simulink model "asbQuadcopter"  (R2021b)
settings: Solver=ode3  StartTime=0  StopTime=200  FixedStep=Ts  RelTol=1e-3  EnableMultiTasking=on
undefined symbols (not defined in the file or in its folder): Command, ft, init, m, s, takeOffDuration, Ts, Vehicle
libraries: simulink x6, aerolibconvert2 x5, aerolibanimutils x3, environmentLibrary x2, SignalEditorBlockLib x2, sensorsLibrary x2, aerolibfltsims x2, aerolibutil x2, vrlib x1
settings Model: Creator=The MathWorks, Inc.  LastModifiedBy=LENOVO
settings SolverCC: AlgebraicLoopSolver=TrustRegion
settings DataIOCC: LimitDataPoints=on  SaveFormat=Array  SaveOutput=off  SignalLogging=off  DSMLogging=off  SaveTime=off  ReturnWorkspaceOutputs=off
settings OptimizationCC: BlockReduction=off  BufferReuse=off  LifeSpan=inf
settings DebuggingCC: AlgebraicLoopMsg=none  ParameterPrecisionLossMsg=none  UnconnectedInputMsg=none  UnconnectedOutputMsg=none  UnconnectedLineMsg=none  AllowSymbolicDim=off  PregeneratedLibrarySubsystemCodeDiagnostic=none  SFUnexpectedBacktrackingDiag=warning  SFNoUnconditionalDefaultTransitionDiag=warning  SFExecutionAtInitializationDiag=none  SFMachineParentedDataDiag=warning  ArithmeticOperatorsInVariantConditions=warning
settings HardwareCC: ProdBitPerPointer=32  ProdBitPerSizeT=32  ProdBitPerPtrDiffT=32  ProdLargestAtomicFloat=None  ProdIntDivRoundTo=Undefined  ProdEndianess=Unspecified  ProdWordSize=32  ProdHWDeviceType=32-bit Generic
settings ModelReferenceCC: PropagateSignalLabelsOutOfModel=off
settings SFSimCC: SimUseLocalCustomCode=off  CustomCodeUndefinedFunction=UseInterfaceOnly
settings RTWCC: RTWUseLocalCustomCode=off
settings CodeAppCC: StateflowObjectComments=on
settings GRTTargetCC: TargetLangStandard=C89/C90 (ANSI)
settings ConfigComp: CovMetricSettings=dw  CovSaveCumulativeToWorkspaceVar=on  CovSaveSingleToWorkspaceVar=on  CovExternalEMLEnable=off  CovSFcnEnable=off

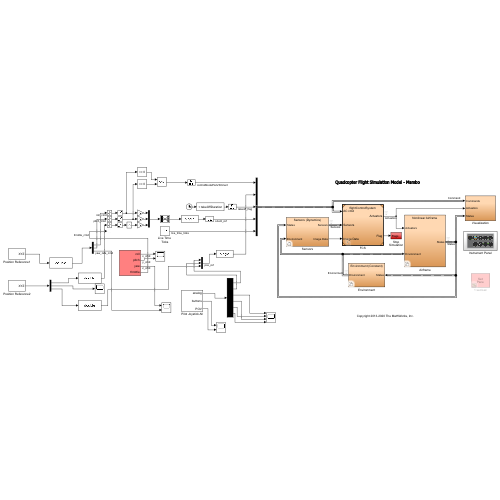
[thumbnail: Simulink's stored preview of the top-level diagram]
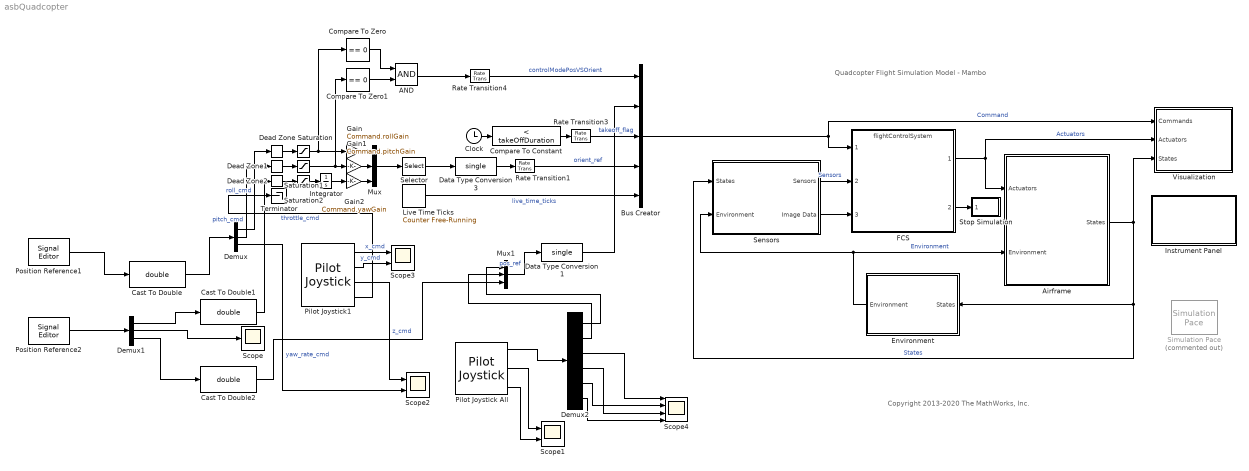
== system asbQuadcopter ==
  note: Quadcopter Flight Simulation Model - Mambo
  note: Copyright 2013-2020 The MathWorks, Inc.
  AND : Logic  AllPortsSameDT=off  OutDataTypeStr=boolean
  Airframe : Subsystem  Variant=on
  Bus Creator : BusCreator  Inputs=5  OutDataTypeStr=Bus: CommandBus  NonVirtualBus=on
  Cast To Double : DataTypeConversion  OutDataTypeStr=double
  Cast To Double1 : DataTypeConversion  OutDataTypeStr=double
  Cast To Double2 : DataTypeConversion  OutDataTypeStr=double
  Clock : Clock
  Compare To Constant : simulink/Logic and Bit Operations/Compare To Constant  relop=<  const=takeOffDuration  OutDataTypeStr=boolean
  Compare To Zero : simulink/Logic and Bit Operations/Compare To Zero  relop===  OutDataTypeStr=boolean
  Compare To Zero1 : simulink/Logic and Bit Operations/Compare To Zero  relop===  OutDataTypeStr=boolean
  Data Type Conversion1 : DataTypeConversion  OutDataTypeStr=single
  Data Type Conversion3 : DataTypeConversion  OutDataTypeStr=single
  Dead Zone : DeadZone  LowerValue=Command.rollDeadZoneStart  UpperValue=Command.rollDeadZoneEnd  SaturateOnIntegerOverflow=on
  Dead Zone1 : DeadZone  LowerValue=Command.pitchDeadZoneStart  UpperValue=Command.pitchDeadZoneEnd  SaturateOnIntegerOverflow=on
  Dead Zone2 : DeadZone  LowerValue=Command.yawDeadZoneStart  UpperValue=Command.yawDeadZoneEnd  SaturateOnIntegerOverflow=on
  Demux : Demux  Outputs=3
  Demux1 : Demux  Outputs=3
  Demux2 : Demux  Outputs=6
  Environment : Subsystem  Variant=on
  FCS : ModelReference  ModelNameDialog=flightControlSystem.slx  SimulationMode=Normal  ModelReferenceVersion=5.0
  Gain : Gain  Gain=Command.rollGain
  Gain1 : Gain  Gain=Command.pitchGain
  Gain2 : Gain  Gain=Command.yawGain
  Instrument Panel : Subsystem
  Integrator : Integrator
  Live Time Ticks : simulink/Sources/Counter Free-Running  NumBits=32  tsamp=Ts
  Mux : Mux  Inputs=3
  Mux1 : Mux  Inputs=3
  Pilot Joystick All : aerolibanimutils/Pilot Joystick  JoystickID=Joystick1  OutputConfiguration=AllOutputs  SampleTime=0.005
  Pilot Joystick1 : aerolibanimutils/Pilot Joystick  JoystickID=Joystick1  OutputConfiguration=FourAxis  SampleTime=Ts
  Position Reference1 : SignalEditorBlockLib/Signal Editor  FileName=positionRef.mat  ActiveScenario=Group1  ActiveSignal=XYZ  IsBus=off  OutputBusObjectStr=Bus: BusObject  SampleTime=Ts  ZeroCross=off  OutputAfterFinalValue=Setting to zero  Unit=inherit  PreserveSignalName=on
  Position Reference2 : SignalEditorBlockLib/Signal Editor  FileName=positionRef.mat  ActiveScenario=Group1  ActiveSignal=XYZ  IsBus=off  OutputBusObjectStr=Bus: BusObject  SampleTime=Ts  ZeroCross=off  OutputAfterFinalValue=Setting to zero  Unit=inherit  PreserveSignalName=on
  Rate Transition1 : RateTransition  OutPortSampleTime=Ts
  Rate Transition3 : RateTransition  OutPortSampleTime=Ts
  Rate Transition4 : RateTransition  OutPortSampleTime=Ts
  Saturation : Saturate  UpperLimit=Command.rollSatUpper  LowerLimit=Command.rollSatLower
  Saturation1 : Saturate  UpperLimit=Command.pitchSatUpper  LowerLimit=Command.pitchSatLower
  Saturation2 : Saturate  UpperLimit=Command.yawSatUpper  LowerLimit=Command.yawSatLower
  Scope : Scope
  Scope1 : Scope  NumInputPorts=2
  Scope2 : Scope  NumInputPorts=2
  Scope3 : Scope  NumInputPorts=2
  Scope4 : Scope  NumInputPorts=4
  Selector : Selector  InputPortWidth=3  IndexOptions=Index vector (dialog)  Indices=[3 2 1]  OutputSizes=1
  Sensors : Subsystem  Variant=on
  Simulation Pace : aerolibanimutils/Simulation Pace  Commented=on  SimulationPace=1  SleepMode=MATLAB Thread  OutputPaceError=off  SampleTime=Ts
      settings: AttributesFormatString=%<SimulationPace> sec/sec
  Stop Simulation : Subsystem
  Terminator : Terminator
  Visualization : Subsystem
  wires:
  Bus Creator/1 -> Visualization/1(Commands), FCS/1  "Command"
  Sensors/1(Sensors) -> FCS/2  "Sensors"
  FCS/1 -> Visualization/2(Actuators), Airframe/1(Actuators)  "Actuators"
  Environment/1(Environment) -> Airframe/2(Environment), Sensors/2(Environment)  "Environment"
  Airframe/1(States) -> Visualization/3(States), Environment/1(States), Sensors/1(States)  "States"
  FCS/2 -> Stop Simulation/1(Flags)
  Sensors/2(Image Data) -> FCS/3
  Rate Transition1/1 -> Bus Creator/4  "orient_ref"
  AND/1 -> Rate Transition4/1
  Gain/1 -> Mux/1
  Dead Zone2/1 -> Saturation2/1
  Live Time Ticks/1 -> Bus Creator/5  "live_time_ticks"
  Saturation/1 -> Compare To Zero/1, Gain/1
  Gain1/1 -> Mux/2
  Selector/1 -> Data Type Conversion3/1
  Dead Zone/1 -> Saturation/1
  Mux/1 -> Selector/1
  Compare To Constant/1 -> Rate Transition3/1
  Demux/1 -> Dead Zone/1  "roll_cmd"
  Rate Transition3/1 -> Bus Creator/3  "takeoff_flag"
  Data Type Conversion3/1 -> Rate Transition1/1
  Gain2/1 -> Mux/3
  Clock/1 -> Compare To Constant/1
  Dead Zone1/1 -> Saturation1/1
  Saturation1/1 -> Compare To Zero1/1, Gain1/1
  Compare To Zero1/1 -> AND/2
  Compare To Zero/1 -> AND/1
  Pilot Joystick1/4 -> Terminator/1  "throttle_cmd"
  Rate Transition4/1 -> Bus Creator/1  "controlModePosVSOrient"
  Saturation2/1 -> Integrator/1
  Integrator/1 -> Gain2/1
  Demux/2 -> Dead Zone1/1  "pitch_cmd"
  Mux1/1 -> Data Type Conversion1/1  "pos_ref"
  Data Type Conversion1/1 -> Bus Creator/2
  Position Reference1/1 -> Cast To Double/1
  Cast To Double/1 -> Demux/1
  Position Reference2/1 -> Demux1/1
  Demux1/1 -> Cast To Double1/1
  Cast To Double1/1 -> Dead Zone2/1
  Pilot Joystick1/3 -> Scope2/1  "z_cmd"
  Demux/3 -> Scope2/2  "yaw_rate_cmd"
  Demux1/2 -> Scope/1
  Demux1/3 -> Cast To Double2/1
  Cast To Double2/1 -> Mux1/3
  Pilot Joystick All/2 -> Scope1/1
  Pilot Joystick All/3 -> Scope1/2
  Pilot Joystick All/1 -> Demux2/1
  Demux2/1 -> Mux1/1
  Demux2/2 -> Mux1/2
  Pilot Joystick1/1 -> Scope3/1  "x_cmd"
  Pilot Joystick1/2 -> Scope3/2  "y_cmd"
  Demux2/3 -> Scope4/1
  Demux2/4 -> Scope4/3
  Demux2/5 -> Scope4/2
  Demux2/6 -> Scope4/4

== system asbQuadcopter/Airframe ==
  note: VSS_VEHICLE = 0 will select linear airframe
      | VSS_VEHICLE = 1 will select nonlnear airframe
  Actuators : Inport
  Environment : Inport  Port=2  OutDataTypeStr=Bus: EnvironmentBus
  Linear Airframe : ModelReference  ModelNameDialog=linearAirframe.slx  SimulationMode=Normal  VariantControl=VSS_VEHICLE_LINEAR  ModelReferenceVersion=5.0
  Nonlinear Airframe : ModelReference  ModelNameDialog=nonlinearAirframe.slx  SimulationMode=Normal  VariantControl=VSS_VEHICLE_NONLINEAR  ModelReferenceVersion=5.0
  States : Outport  OutDataTypeStr=Bus: StatesBus  VectorParamsAs1DForOutWhenUnconnected=off

== system asbQuadcopter/Environment ==
  note: VSS_ENVIRONMENT = 0 will select constant environment variables
      | VSS_ENVIRONMENT = 1 will select environment variables depending on position
  States : Inport  OutDataTypeStr=Bus: StatesBus
  Environment (Constant) : environmentLibrary/Environment (Constant)  SystemSampleTime=-1  VariantControl=VSS_ENVIRONMENT_CST  VariantActivationTime=update diagram  Latency=0  AutoFrameSizeCalculation=off
  Environment (Variable) : environmentLibrary/Environment (Variable)  SystemSampleTime=-1  VariantControl=VSS_ENVIRONMENT_VARIABLE  VariantActivationTime=update diagram  Latency=0  AutoFrameSizeCalculation=off
  Environment : Outport  OutDataTypeStr=Bus: EnvironmentBus  VectorParamsAs1DForOutWhenUnconnected=off

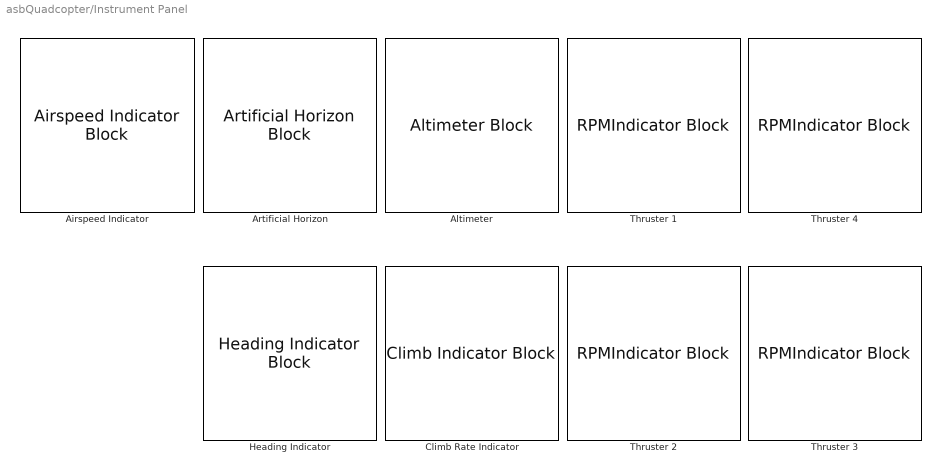
== system asbQuadcopter/Instrument Panel ==
  Airspeed Indicator : AirspeedIndicatorBlock  LabelPosition=Hide  ScaleMin=0  ScaleMax=18
  Altimeter : AltimeterBlock  LabelPosition=Hide
  Artificial Horizon : ArtificialHorizonBlock  LabelPosition=Hide
  Climb Rate Indicator : ClimbIndicatorBlock  LabelPosition=Hide  ScaleMax=1000
  Heading Indicator : HeadingIndicatorBlock  LabelPosition=Hide
  Thruster {1..4} (4 alike) : RPMIndicatorBlock  LabelPosition=Hide

== system asbQuadcopter/Sensors ==
  note: VSS_SENSORS = 0 will select feedthrough sensors
      | VSS_SENSORS = 1 will select dynamics sensors with noise
  States : Inport
  Environment : Inport  Port=2
  Sensors (Dynamics) : sensorsLibrary/Sensors (Dynamics)  SystemSampleTime=-1  VariantControl=VSS_SENSORS_DYNAMICS  VariantActivationTime=update diagram  Latency=0  AutoFrameSizeCalculation=off
  Sensors (Feedthrough) : sensorsLibrary/Sensors (Feedthrough)  SystemSampleTime=-1  VariantControl=VSS_SENSORS_FEEDTHROUGH  VariantActivationTime=update diagram  Latency=0  AutoFrameSizeCalculation=off
  Sensors : Outport  VectorParamsAs1DForOutWhenUnconnected=off
  Image Data : Outport  Port=2  VectorParamsAs1DForOutWhenUnconnected=off

== system asbQuadcopter/Stop Simulation ==
  Flags : Inport  OutDataTypeStr=uint8
  Compare To Zero : simulink/Logic and Bit Operations/Compare To Zero  relop=>  OutDataTypeStr=boolean
  Flag has been triggered : Assertion
  Logical Operator : Logic  Operator=NOT  AllPortsSameDT=off  OutDataTypeStr=boolean
  wires:
  Flags/1 -> Compare To Zero/1
  Logical Operator/1 -> Flag has been triggered/1
  Compare To Zero/1 -> Logical Operator/1

== system asbQuadcopter/Visualization ==
  Commands : Inport
  Actuators : Inport  Port=2
  States : Inport  Port=3
  "Actuators " : InportShadow  Port=2
  Extract Flight Instruments : Subsystem
  "States " : InportShadow  Port=3
  Visualization : Subsystem  Variant=on
  wires:
  Actuators/1 -> Extract Flight Instruments/1(Actuators)
  States/1 -> Extract Flight Instruments/2(States)
  Commands/1 -> Visualization/2(Commands)
  "Actuators "/1 -> Visualization/3(Actuators)
  "States "/1 -> Visualization/1(States)

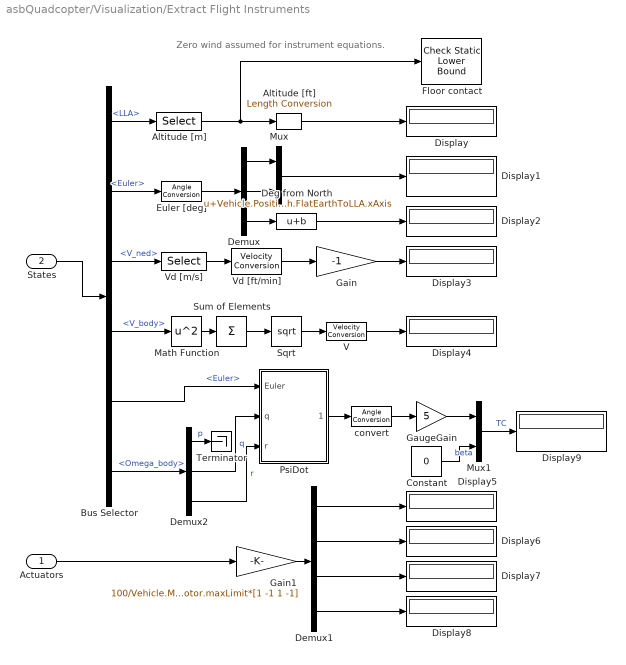
== system asbQuadcopter/Visualization/Extract Flight Instruments ==
  note: Zero wind assumed for instrument equations.
  Actuators : Inport
  States : Inport  Port=2
  Altitude [ft] : aerolibconvert2/Length Conversion  IU=m  OU=ft
  Altitude [m] : Selector  InputPortWidth=3  IndexOptions=Index vector (dialog)  Indices=[3]  OutputSizes=1
  Bus Selector : BusSelector  OutputSignals=LLA,Euler,V_ned,V_body,Euler,Omega_body
  Constant : Constant  Value=0
  Deg from North : Bias  Bias=Vehicle.PositionOnEarth.FlatEarthToLLA.xAxis
  Demux : Demux  Outputs=3
  Demux1 : Demux
  Demux2 : Demux  Outputs=3
  Display{,1..9} (10 alike) : Display
  Euler [deg] : aerolibconvert2/Angle Conversion  IU=rad  OU=deg
  Floor contact : simulink/Model Verification/Check Static  Lower Bound  Description=init.posLLA(3) <= u  min=init.posLLA(3)  min_included=on  enabled=on  stopWhenAssertionFail=on  export=off  icon=graphic
  Gain : Gain  Gain=-1
  Gain1 : Gain  Gain=100/Vehicle.Motor.maxLimit*[1 -1 1 -1]
  GaugeGain : Gain  Gain=5
  Math Function : Math  Operator=square  SignedPower=on  SaturateOnIntegerOverflow=on
  Mux : Mux  Inputs=2
  Mux1 : Mux  Inputs=2
  PsiDot : Subsystem
  Sqrt : Sqrt  SaturateOnIntegerOverflow=on
  Sum of Elements : Sum  Inputs=+
  Terminator : Terminator
  V : aerolibconvert2/Velocity Conversion  IU=m/s  OU=kts
  Vd [ft/min] : aerolibconvert2/Velocity Conversion  IU=m/s  OU=ft/min
  Vd [m/s] : Selector  InputPortWidth=3  IndexOptions=Index vector (dialog)  Indices=[3]  OutputSizes=1
  convert : aerolibconvert2/Angle Conversion  IU=rad  OU=deg
  wires:
  Bus Selector/1 -> Altitude [m]/1  "<LLA>"
  Altitude [m]/1 -> Floor contact/1, Altitude [ft]/1
  States/1 -> Bus Selector/1
  Altitude [ft]/1 -> Display/1
  Bus Selector/2 -> Euler [deg]/1  "<Euler>"
  Euler [deg]/1 -> Demux/1
  Demux/1 -> Mux/1
  Demux/2 -> Mux/2
  Mux/1 -> Display1/1
  Deg from North/1 -> Display2/1
  Bus Selector/3 -> Vd [m/s]/1  "<V_ned>"
  Vd [m/s]/1 -> Vd [ft/min]/1
  Vd [ft/min]/1 -> Gain/1
  Gain/1 -> Display3/1
  Math Function/1 -> Sum of Elements/1
  Sum of Elements/1 -> Sqrt/1
  Bus Selector/4 -> Math Function/1  "<V_body>"
  Sqrt/1 -> V/1
  V/1 -> Display4/1
  Gain1/1 -> Demux1/1
  Demux1/1 -> Display5/1
  Demux1/2 -> Display6/1
  Demux1/3 -> Display7/1
  Demux1/4 -> Display8/1
  Actuators/1 -> Gain1/1
  Demux/3 -> Deg from North/1
  Mux1/1 -> Display9/1  "TC"
  Constant/1 -> Mux1/2  "beta"
  Bus Selector/6 -> Demux2/1  "<Omega_body>"
  Demux2/1 -> Terminator/1  "p"
  Demux2/2 -> PsiDot/2(q)  "q"
  Demux2/3 -> PsiDot/3(r)  "r"
  PsiDot/1(psi_dot) -> convert/1
  convert/1 -> GaugeGain/1
  GaugeGain/1 -> Mux1/1
  Bus Selector/5 -> PsiDot/1(Euler)  "<Euler>"

== system asbQuadcopter/Visualization/Visualization ==
  note: VSS_VISUALIZATION = 0 will select scopes as means to visualie variables/states
      | VSS_VISUALIZATION = 1 will send select states in a variable to the workspace
      | VSS_VISUALIZATION = 2 will use FlightGear as visualization
      | VSS_VISUALIZATION = 3 will use a Simulink 3D interface
  States : Inport  OutDataTypeStr=Bus: StatesBus
  Commands : Inport  Port=2  OutDataTypeStr=Bus: CommandBus
  Actuators : Inport  Port=3
  FlightGear : Subsystem  VariantControl=VSS_VISUALIZATION_FLIGHTGEAR
      mask init:
      | visualizationFlightGearVars;
  Scopes : Subsystem  VariantControl=VSS_VISUALIZATION_SCOPES
  Simulink 3D : Subsystem  VariantControl=VSS_VISUALIZATION_SL3D
      mask init:
      | visualizationFlightGearVars;
  Workspace : Subsystem  VariantControl=VSS_VISUALIZATION_WORKSPACE

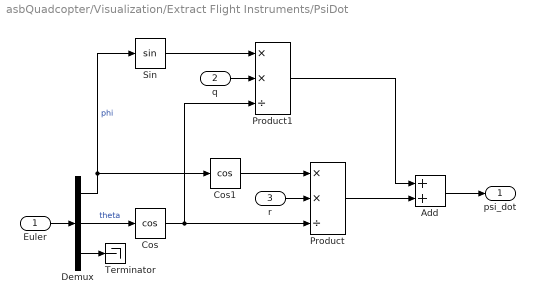
== system asbQuadcopter/Visualization/Extract Flight Instruments/PsiDot ==
  Euler : Inport
  q : Inport  Port=2
  r : Inport  Port=3
  Add : Sum
  Cos : Trigonometry  Operator=cos
  Cos1 : Trigonometry  Operator=cos
  Demux : Demux  Outputs=3
  Product : Product  Inputs=**/
  Product1 : Product  Inputs=**/
  Sin : Trigonometry
  Terminator : Terminator
  psi_dot : Outport
  wires:
  Demux/2 -> Cos/1  "theta"
  Add/1 -> psi_dot/1
  Cos/1 -> Product/3, Product1/3
  q/1 -> Product1/2
  r/1 -> Product/2
  Product1/1 -> Add/1
  Product/1 -> Add/2
  Demux/1 -> Cos1/1, Sin/1  "phi"
  Sin/1 -> Product1/1
  Cos1/1 -> Product/1
  Demux/3 -> Terminator/1
  Euler/1 -> Demux/1

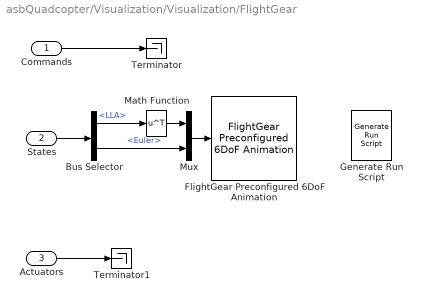
== system asbQuadcopter/Visualization/Visualization/FlightGear ==
  Commands : Inport
  States : Inport  Port=2
  Actuators : Inport  Port=3
  Bus Selector : BusSelector  OutputSignals=LLA,Euler
  FlightGear Preconfigured 6DoF Animation : aerolibfltsims/FlightGear Preconfigured 6DoF Animation  xFlightGearVersion=v2019.1  DestinationIpAddress=127.0.0.1  DestinationPort=Visualization.FlightGear.SixDOF.destinationPort  SampleTime=Ts  packetVersion=24
  Generate Run Script : aerolibfltsims/Generate Run Script  Architecture=Default  dataFlow=Send  GeometryModelName=Model  AirportId=KSFO  RunwayId=10L  InitialAltitude=Visualization.FlightGear.generateRunScript.initialAltitude  InitialHeading=Visualization.FlightGear.generateRunScript.initialHeading  OffsetDistance=Visualization.FlightGear.generateRunScript.offsetDistance  OffsetAzimuth=Visualization.FlightGear.generateRunScript.offsetAzimuth  InstallScenery=off  DisableShaders=off  OriginAddress=127.0.0.1  DestinationPort=Visualization.FlightGear.generateRunScript.destinationPort  OriginPort=5505  LocalAddress=127.0.0.1  OutputFileName=runfg.bat  FlightGearBaseDirectory=C:\Program Files\FlightGear
  Math Function : Math  Operator=transpose  SignedPower=on  SaturateOnIntegerOverflow=on
  Mux : Mux  Inputs=2
  Terminator : Terminator
  Terminator1 : Terminator
  wires:
  States/1 -> Bus Selector/1
  Bus Selector/2 -> Mux/2  "<Euler>"
  Mux/1 -> FlightGear Preconfigured 6DoF Animation/1
  Commands/1 -> Terminator/1
  Actuators/1 -> Terminator1/1
  Bus Selector/1 -> Math Function/1  "<LLA>"
  Math Function/1 -> Mux/1

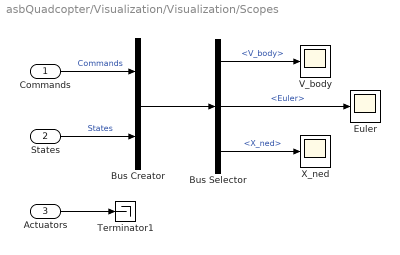
== system asbQuadcopter/Visualization/Visualization/Scopes ==
  Commands : Inport
  States : Inport  Port=2
  Actuators : Inport  Port=3
  Bus Creator : BusCreator  Inputs=2
  Bus Selector : BusSelector  OutputSignals=States.V_body,States.Euler,States.X_ned
  Euler : Scope
  Terminator1 : Terminator
  V_body : Scope
  X_ned : Scope
  wires:
  Commands/1 -> Bus Creator/1  "Commands"
  States/1 -> Bus Creator/2  "States"
  Bus Creator/1 -> Bus Selector/1
  Bus Selector/1 -> V_body/1  "<V_body>"
  Bus Selector/2 -> Euler/1  "<Euler>"
  Bus Selector/3 -> X_ned/1  "<X_ned>"
  Actuators/1 -> Terminator1/1

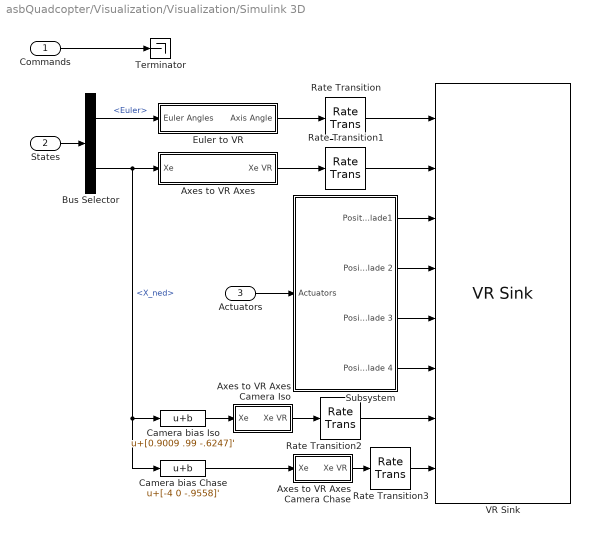
== system asbQuadcopter/Visualization/Visualization/Simulink 3D ==
  Commands : Inport
  States : Inport  Port=2
  Actuators : Inport  Port=3
  Axes to VR Axes : Subsystem
  Axes to VR Axes Camera Chase : Subsystem
  Axes to VR Axes Camera Iso : Subsystem
  Bus Selector : BusSelector  OutputSignals=Euler,X_ned
  Camera bias Chase : Bias  Bias=[-4 0 -.9558]'
  Camera bias Iso : Bias  Bias=[0.9009 .99 -.6247]'
  Euler to VR : Subsystem
  Rate Transition{,1..3} (4 alike) : RateTransition
  Subsystem : Subsystem
  Terminator : Terminator
  VR Sink : vrlib/VR Sink  InstantiateOnLoad=on  SampleTime=12*Ts  ViewEnable=on  RemoteChange=off  RemoteView=off  FieldsWritten=QuadBody.rotation.4.1.1.double#QuadBody.translation.3.1.1.double#Blade1.rotation.4.1.1.double#Blade2.rotation.4.1.1.double#Blade3.rotation.4.1.1.double#Blade4.rotation.4.1.1.double#IsoNoRotation.position.3.1.1.double#OnQuadNoRotation.position.3.1.1.double  WorldFileName=asbQuadcopterWorld.wrl  AutoView=on  VideoDimensions=[]  AllowVariableSize=off
  wires:
  Commands/1 -> Terminator/1
  Euler to VR/1(Axis Angle) -> Rate Transition/1
  Axes to VR Axes/1(Xe VR) -> Rate Transition1/1
  Bus Selector/1 -> Euler to VR/1(Euler Angles)  "<Euler>"
  Bus Selector/2 -> Camera bias Chase/1, Camera bias Iso/1, Axes to VR Axes/1(Xe)  "<X_ned>"
  States/1 -> Bus Selector/1
  Actuators/1 -> Subsystem/1(Actuators)
  Axes to VR Axes Camera Iso/1(Xe VR) -> Rate Transition2/1
  Camera bias Iso/1 -> Axes to VR Axes Camera Iso/1(Xe)
  Rate Transition/1 -> VR Sink/1
  Rate Transition1/1 -> VR Sink/2
  Subsystem/1(Position Blade1) -> VR Sink/3
  Subsystem/2(Position Blade 2) -> VR Sink/4
  Subsystem/3(Position Blade 3) -> VR Sink/5
  Subsystem/4(Position Blade 4) -> VR Sink/6
  Rate Transition2/1 -> VR Sink/7
  Axes to VR Axes Camera Chase/1(Xe VR) -> Rate Transition3/1
  Rate Transition3/1 -> VR Sink/8
  Camera bias Chase/1 -> Axes to VR Axes Camera Chase/1(Xe)

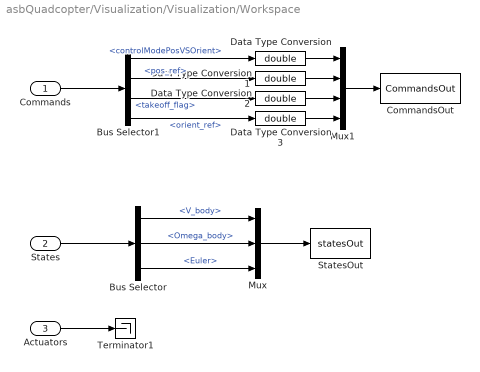
== system asbQuadcopter/Visualization/Visualization/Workspace ==
  Commands : Inport
  States : Inport  Port=2
  Actuators : Inport  Port=3
  Bus Selector : BusSelector  OutputSignals=V_body,Omega_body,Euler
  Bus Selector1 : BusSelector  OutputSignals=controlModePosVSOrient,pos_ref,takeoff_flag,orient_ref
  CommandsOut : ToWorkspace  VariableName=CommandsOut  SaveFormat=Structure With Time  SampleTime=-1
  Data Type Conversion{,1..3} (4 alike) : DataTypeConversion  OutDataTypeStr=double
  Mux : Mux  Inputs=3
  Mux1 : Mux
  StatesOut : ToWorkspace  VariableName=statesOut  SaveFormat=Structure With Time  SampleTime=-1
  Terminator1 : Terminator
  wires:
  States/1 -> Bus Selector/1
  Bus Selector/2 -> Mux/2  "<Omega_body>"
  Bus Selector/3 -> Mux/3  "<Euler>"
  Bus Selector/1 -> Mux/1  "<V_body>"
  Mux/1 -> StatesOut/1
  Commands/1 -> Bus Selector1/1
  Bus Selector1/2 -> Data Type Conversion1/1  "<pos_ref>"
  Bus Selector1/1 -> Data Type Conversion/1  "<controlModePosVSOrient>"
  Mux1/1 -> CommandsOut/1
  Bus Selector1/4 -> Data Type Conversion3/1  "<orient_ref>"
  Bus Selector1/3 -> Data Type Conversion2/1  "<takeoff_flag>"
  Actuators/1 -> Terminator1/1
  Data Type Conversion/1 -> Mux1/1
  Data Type Conversion1/1 -> Mux1/2
  Data Type Conversion2/1 -> Mux1/3
  Data Type Conversion3/1 -> Mux1/4

== system asbQuadcopter/Visualization/Visualization/Simulink 3D/Axes to VR Axes ==
  Xe : Inport
  Demux : Demux  Outputs=3
      settings: DisplayOption=none
  Mux : Mux  Inputs=3
  rad-->deg1 : Gain  Gain=-1  SaturateOnIntegerOverflow=on  OutDataTypeStr=Inherit: Same as input  ParamDataTypeStr=Inherit: Same as input
  Xe VR : Outport  VectorParamsAs1DForOutWhenUnconnected=off
  wires:
  Xe/1 -> Demux/1
  Demux/1 -> Mux/1
  Demux/3 -> rad-->deg1/1
  Mux/1 -> Xe VR/1
  rad-->deg1/1 -> Mux/2
  Demux/2 -> Mux/3

== system asbQuadcopter/Visualization/Visualization/Simulink 3D/Axes to VR Axes Camera Chase ==
  Xe : Inport
  Demux : Demux  Outputs=3
      settings: DisplayOption=none
  Mux : Mux  Inputs=3
  rad-->deg1 : Gain  Gain=-1  SaturateOnIntegerOverflow=on  OutDataTypeStr=Inherit: Same as input  ParamDataTypeStr=Inherit: Same as input
  Xe VR : Outport  VectorParamsAs1DForOutWhenUnconnected=off
  wires:
  Xe/1 -> Demux/1
  Demux/1 -> Mux/1
  Demux/3 -> rad-->deg1/1
  Mux/1 -> Xe VR/1
  rad-->deg1/1 -> Mux/2
  Demux/2 -> Mux/3

== system asbQuadcopter/Visualization/Visualization/Simulink 3D/Axes to VR Axes Camera Iso ==
  Xe : Inport
  Demux : Demux  Outputs=3
      settings: DisplayOption=none
  Mux : Mux  Inputs=3
  rad-->deg1 : Gain  Gain=-1  SaturateOnIntegerOverflow=on  OutDataTypeStr=Inherit: Same as input  ParamDataTypeStr=Inherit: Same as input
  Xe VR : Outport  VectorParamsAs1DForOutWhenUnconnected=off
  wires:
  Demux/2 -> Mux/3
  rad-->deg1/1 -> Mux/2
  Mux/1 -> Xe VR/1
  Demux/3 -> rad-->deg1/1
  Demux/1 -> Mux/1
  Xe/1 -> Demux/1

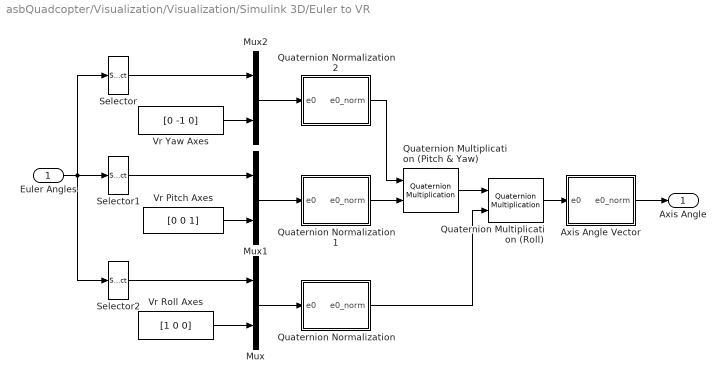
== system asbQuadcopter/Visualization/Visualization/Simulink 3D/Euler to VR ==
  Euler Angles : Inport
  Axis Angle Vector : Subsystem
  Mux : Mux  Inputs=2
  Mux1 : Mux  Inputs=2
  Mux2 : Mux  Inputs=2
  Quaternion Multiplication (Pitch & Yaw) : aerolibutil/Quaternion Multiplication
  Quaternion Multiplication (Roll) : aerolibutil/Quaternion Multiplication
  Quaternion Normalization : Subsystem
  Quaternion Normalization1 : Subsystem
  Quaternion Normalization2 : Subsystem
  Selector : Selector  InputPortWidth=3  IndexOptions=Index vector (dialog)  Indices=[3]  OutputSizes=1
  Selector1 : Selector  InputPortWidth=3  IndexOptions=Index vector (dialog)  Indices=[2]  OutputSizes=1
  Selector2 : Selector  InputPortWidth=3  IndexOptions=Index vector (dialog)  Indices=[1]  OutputSizes=1
  Vr Pitch Axes : Constant  Value=[0 0 1]
  Vr Roll Axes : Constant  Value=[1 0 0]
  Vr Yaw Axes : Constant  Value=[0 -1 0]
  Axis Angle : Outport  VectorParamsAs1DForOutWhenUnconnected=off
  wires:
  Quaternion Multiplication (Roll)/1 -> Axis Angle Vector/1(e0)
  Axis Angle Vector/1(e0_norm) -> Axis Angle/1
  Quaternion Normalization/1(e0_norm) -> Quaternion Multiplication (Roll)/2
  Quaternion Normalization2/1(e0_norm) -> Quaternion Multiplication (Pitch & Yaw)/1
  Quaternion Normalization1/1(e0_norm) -> Quaternion Multiplication (Pitch & Yaw)/2
  Mux2/1 -> Quaternion Normalization2/1(e0)
  Mux1/1 -> Quaternion Normalization1/1(e0)
  Mux/1 -> Quaternion Normalization/1(e0)
  Selector/1 -> Mux2/1
  Vr Yaw Axes/1 -> Mux2/2
  Selector1/1 -> Mux1/1
  Vr Pitch Axes/1 -> Mux1/2
  Selector2/1 -> Mux/1
  Vr Roll Axes/1 -> Mux/2
  Euler Angles/1 -> Selector2/1, Selector1/1, Selector/1
  Quaternion Multiplication (Pitch & Yaw)/1 -> Quaternion Multiplication (Roll)/1

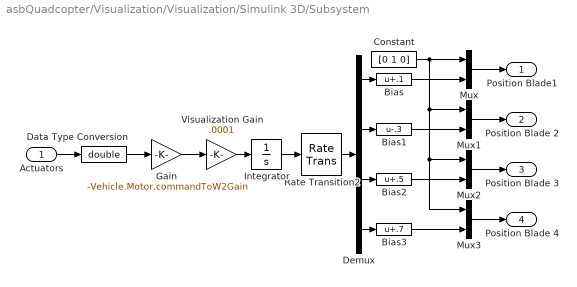
== system asbQuadcopter/Visualization/Visualization/Simulink 3D/Subsystem ==
  Actuators : Inport
  Bias : Bias  Bias=.1
  Bias1 : Bias  Bias=-.3
  Bias2 : Bias  Bias=.5
  Bias3 : Bias  Bias=.7
  Constant : Constant  Value=[0 1 0]
  Data Type Conversion : DataTypeConversion  OutDataTypeStr=double
  Demux : Demux
  Gain : Gain  Gain=-Vehicle.Motor.commandToW2Gain
  Integrator : Integrator  InitialCondition="[.1  .2 -.3 -.4]"  WrapState=on  WrappedStateUpperValue=2*pi  WrappedStateLowerValue=-2*pi
  Mux{,1..3} (4 alike) : Mux  Inputs=2
  Rate Transition2 : RateTransition
  Visualization Gain : Gain  Gain=.0001
  Position Blade1 : Outport  VectorParamsAs1DForOutWhenUnconnected=off
  Position Blade 2 : Outport  Port=2  VectorParamsAs1DForOutWhenUnconnected=off
  Position Blade 3 : Outport  Port=3  VectorParamsAs1DForOutWhenUnconnected=off
  Position Blade 4 : Outport  Port=4  VectorParamsAs1DForOutWhenUnconnected=off
  wires:
  Bias3/1 -> Mux3/2
  Mux3/1 -> Position Blade 4/1
  Bias1/1 -> Mux1/2
  Bias2/1 -> Mux2/2
  Demux/2 -> Bias1/1
  Visualization Gain/1 -> Integrator/1
  Constant/1 -> Mux3/1, Mux2/1, Mux1/1, Mux/1
  Mux1/1 -> Position Blade 2/1
  Mux2/1 -> Position Blade 3/1
  Data Type Conversion/1 -> Gain/1
  Integrator/1 -> Rate Transition2/1
  Mux/1 -> Position Blade1/1
  Gain/1 -> Visualization Gain/1
  Demux/3 -> Bias2/1
  Bias/1 -> Mux/2
  Actuators/1 -> Data Type Conversion/1
  Demux/4 -> Bias3/1
  Rate Transition2/1 -> Demux/1
  Demux/1 -> Bias/1

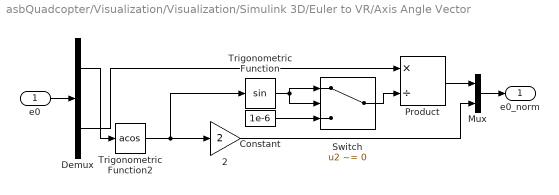
== system asbQuadcopter/Visualization/Visualization/Simulink 3D/Euler to VR/Axis Angle Vector ==
  e0 : Inport
  2 : Gain  Gain=2  SaturateOnIntegerOverflow=on  OutDataTypeStr=Inherit: Same as input  ParamDataTypeStr=Inherit: Same as input
  Constant : Constant  Value=1e-6
  Demux : Demux  Outputs=[1 3 ]
      settings: DisplayOption=none
  Mux : Mux  Inputs=2
  Product : Product  Inputs=*/  InputSameDT=on  SaturateOnIntegerOverflow=on  OutDataTypeStr=Inherit: Same as first input
  Switch : Switch  Criteria=u2 ~= 0
  Trigonometric Function : Trigonometry
  Trigonometric Function2 : Trigonometry  Operator=acos
  e0_norm : Outport  VectorParamsAs1DForOutWhenUnconnected=off
  wires:
  Demux/1 -> Trigonometric Function2/1
  Demux/2 -> Product/1
  Mux/1 -> e0_norm/1
  Product/1 -> Mux/1
  2/1 -> Mux/2
  Trigonometric Function/1 -> Switch/1, Switch/2
  Trigonometric Function2/1 -> Trigonometric Function/1, 2/1
  e0/1 -> Demux/1
  Constant/1 -> Switch/3
  Switch/1 -> Product/2

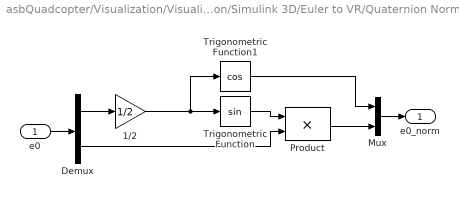
== system asbQuadcopter/Visualization/Visualization/Simulink 3D/Euler to VR/Quaternion Normalization ==
  e0 : Inport
  1/2 : Gain  Gain=1/2  SaturateOnIntegerOverflow=on  OutDataTypeStr=Inherit: Same as input  ParamDataTypeStr=Inherit: Same as input
  Demux : Demux  Outputs=[1 3]
      settings: DisplayOption=none
  Mux : Mux  Inputs=2
  Product : Product  InputSameDT=on  SaturateOnIntegerOverflow=on  OutDataTypeStr=Inherit: Same as first input
  Trigonometric Function : Trigonometry
  Trigonometric Function1 : Trigonometry  Operator=cos
  e0_norm : Outport  VectorParamsAs1DForOutWhenUnconnected=off
  wires:
  Trigonometric Function1/1 -> Mux/1
  Demux/2 -> Product/2
  Demux/1 -> 1/2/1
  Mux/1 -> e0_norm/1
  Product/1 -> Mux/2
  Trigonometric Function/1 -> Product/1
  1/2/1 -> Trigonometric Function1/1, Trigonometric Function/1
  e0/1 -> Demux/1

== system asbQuadcopter/Visualization/Visualization/Simulink 3D/Euler to VR/Quaternion Normalization1 ==
  e0 : Inport
  1/2 : Gain  Gain=1/2  SaturateOnIntegerOverflow=on  OutDataTypeStr=Inherit: Same as input  ParamDataTypeStr=Inherit: Same as input
  Demux : Demux  Outputs=[1 3]
      settings: DisplayOption=none
  Mux : Mux  Inputs=2
  Product : Product  InputSameDT=on  SaturateOnIntegerOverflow=on  OutDataTypeStr=Inherit: Same as first input
  Trigonometric Function : Trigonometry
  Trigonometric Function1 : Trigonometry  Operator=cos
  e0_norm : Outport  VectorParamsAs1DForOutWhenUnconnected=off
  wires:
  e0/1 -> Demux/1
  1/2/1 -> Trigonometric Function/1, Trigonometric Function1/1
  Trigonometric Function/1 -> Product/1
  Product/1 -> Mux/2
  Mux/1 -> e0_norm/1
  Demux/1 -> 1/2/1
  Demux/2 -> Product/2
  Trigonometric Function1/1 -> Mux/1

== system asbQuadcopter/Visualization/Visualization/Simulink 3D/Euler to VR/Quaternion Normalization2 ==
  e0 : Inport
  1/2 : Gain  Gain=1/2  SaturateOnIntegerOverflow=on  OutDataTypeStr=Inherit: Same as input  ParamDataTypeStr=Inherit: Same as input
  Demux : Demux  Outputs=[1 3]
      settings: DisplayOption=none
  Mux : Mux  Inputs=2
  Product : Product  InputSameDT=on  SaturateOnIntegerOverflow=on  OutDataTypeStr=Inherit: Same as first input
  Trigonometric Function : Trigonometry
  Trigonometric Function1 : Trigonometry  Operator=cos
  e0_norm : Outport  VectorParamsAs1DForOutWhenUnconnected=off
  wires:
  Trigonometric Function1/1 -> Mux/1
  Demux/2 -> Product/2
  Demux/1 -> 1/2/1
  Mux/1 -> e0_norm/1
  Product/1 -> Mux/2
  Trigonometric Function/1 -> Product/1
  1/2/1 -> Trigonometric Function1/1, Trigonometric Function/1
  e0/1 -> Demux/1
